simulink model "parallel_8_prediction"  (R2022a)
settings: Solver=FixedStepDiscrete  StartTime=0.0  StopTime=10.0  RelTol=1e-3
undefined symbols (not defined in the file or in its folder): f_c, L_d, L_q, L_x, L_y, p, psi_pm, R_ph
libraries: hdlsllib x5
(part 1 of 2)
settings Model: DataTypeOverride=Off  Creator=Andre Merx  LastModifiedBy=Andre Merx
settings SolverCC: AlgebraicLoopSolver=TrustRegion
settings DataIOCC: LimitDataPoints=on  SaveOutput=off  SaveTime=off
settings OptimizationCC: BlockReduction=off  ConditionallyExecuteInputs=off  DefaultParameterBehavior=Inlined  LifeSpan=inf
settings DebuggingCC: AlgebraicLoopMsg=error  SingleTaskRateTransMsg=error  UnconnectedInputMsg=warning  UnconnectedOutputMsg=warning  UnconnectedLineMsg=warning  AllowSymbolicDim=off  StrictBusMsg=ErrorOnBusTreatedAsVector  SFUnexpectedBacktrackingDiag=warning  SFNoUnconditionalDefaultTransitionDiag=warning  SFExecutionAtInitializationDiag=none  SFMachineParentedDataDiag=warning  ArithmeticOperatorsInVariantConditions=warning
settings HardwareCC: ProdBitPerPointer=32  ProdBitPerSizeT=32  ProdBitPerPtrDiffT=32  ProdLargestAtomicFloat=None  ProdIntDivRoundTo=Undefined  ProdEndianess=Unspecified  ProdWordSize=32  ProdHWDeviceType=ASIC/FPGA->ASIC/FPGA  ProdEqTarget=off
settings SFSimCC: SimUseLocalCustomCode=off  CustomCodeUndefinedFunction=UseInterfaceOnly
settings RTWCC: RTWUseLocalCustomCode=off
settings CodeAppCC: StateflowObjectComments=on
settings GRTTargetCC: TargetLangStandard=C89/C90 (ANSI)
settings ConfigComp: CovScope=ReferencedModels  CovMetricSettings=dw  CovSaveCumulativeToWorkspaceVar=on  CovSaveSingleToWorkspaceVar=on  CovExternalEMLEnable=off  CovSFcnEnable=off

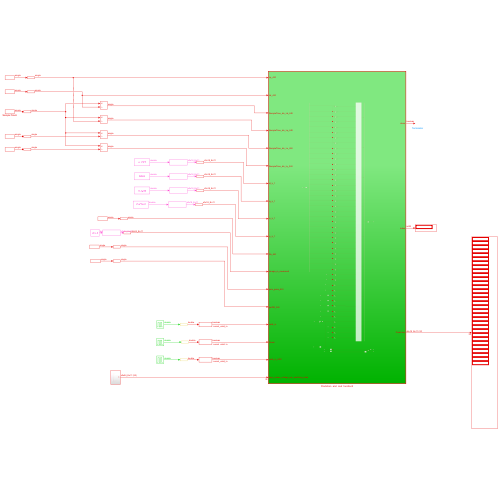
[thumbnail: Simulink's stored preview of the top-level diagram]
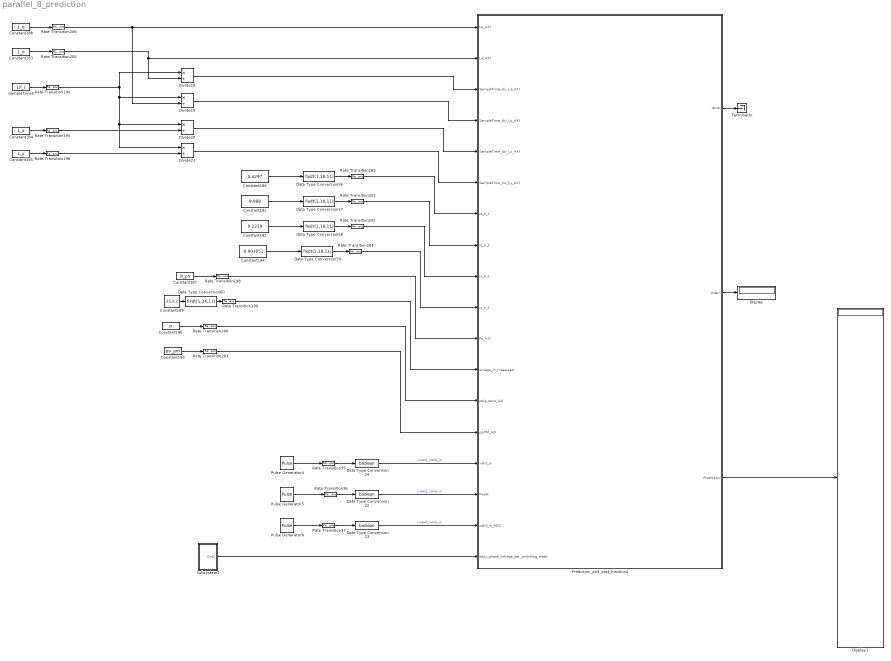
== system parallel_8_prediction ==
  Constant183 : Constant  Value=L_d  OutDataTypeStr=single  SampleTime=-1
  Constant184 : Constant  Value=L_x  OutDataTypeStr=single  SampleTime=-1
  Constant185 : Constant  Value=L_y  OutDataTypeStr=single  SampleTime=-1
  Constant186 : Constant  Value=0.4297
  Constant187 : Constant  Value=R_ph  OutDataTypeStr=single  SampleTime=-1
  Constant188 : Constant  Value=L_q  OutDataTypeStr=single  SampleTime=-1
  Constant189 : Constant  Value=313.3
  Constant190 : Constant  Value=p  OutDataTypeStr=single  SampleTime=-1
  Constant191 : Constant  Value=9.988
  Constant192 : Constant  Value=0.2219
  Constant193 : Constant  Value=psi_pm  OutDataTypeStr=single  SampleTime=-1
  Constant194 : Constant  Value=-0.003051
  Data Type Conversion22 : DataTypeConversion  OutDataTypeStr=boolean  SaturateOnIntegerOverflow=off  RndMeth=Floor
  Data Type Conversion23 : DataTypeConversion  OutDataTypeStr=boolean  SaturateOnIntegerOverflow=off  RndMeth=Floor
  Data Type Conversion24 : DataTypeConversion  OutDataTypeStr=boolean  SaturateOnIntegerOverflow=off  RndMeth=Floor
  Data Type Conversion{56..59} (4 alike) : DataTypeConversion  OutDataTypeStr=fixdt(1,18,11)  SaturateOnIntegerOverflow=off  RndMeth=Floor
  Data Type Conversion60 : DataTypeConversion  OutDataTypeStr=fixdt(1,24,11)  SaturateOnIntegerOverflow=off  RndMeth=Floor
  Display : Display
  Display1 : Display
  Divide{18..21} (4 alike) : Product  Inputs=*/  RndMeth=Zero  SaturateOnIntegerOverflow=on
  Prediction_and_cost_function2 : Subsystem  TreatAsAtomicUnit=on
  Pulse Generator4 : DiscretePulseGenerator  PulseType=Time based  Period=1/f_c
  Pulse Generator5 : DiscretePulseGenerator  PulseType=Time based  Period=1/f_c
  Pulse Generator6 : DiscretePulseGenerator  PulseType=Time based  Period=1/f_c
  Rate Transition{35..37,193..196,198..206} (16 alike) : RateTransition  OutPortSampleTime=Rt
  SampleTime5 : Constant  Value=1/f_c  OutDataTypeStr=single  SampleTime=-1
  Subsystem2 : Subsystem
  Terminator : Terminator
  wires:
  Data Type Conversion60/1 -> Rate Transition199/1
  Rate Transition199/1 -> Prediction_and_cost_function2/12(omega_m_measured)
  Constant194/1 -> Data Type Conversion59/1
  Constant188/1 -> Rate Transition206/1
  Rate Transition201/1 -> Prediction_and_cost_function2/8(iq_k_1)
  Data Type Conversion59/1 -> Rate Transition204/1
  Constant190/1 -> Rate Transition200/1
  Subsystem2/1(Out1) -> Prediction_and_cost_function2/18(dqxy_phase_voltage_per_switching_state)
  Rate Transition205/1 -> Divide18/2, Prediction_and_cost_function2/2(Ld_AXI)
  Data Type Conversion58/1 -> Rate Transition202/1
  Rate Transition195/1 -> Divide20/2
  SampleTime5/1 -> Rate Transition194/1
  Constant186/1 -> Data Type Conversion56/1
  Data Type Conversion57/1 -> Rate Transition201/1
  Divide20/1 -> Prediction_and_cost_function2/5(SampleTime_div_Lx_AXI)
  Constant187/1 -> Rate Transition198/1
  Rate Transition203/1 -> Prediction_and_cost_function2/14(psiPM_AXI)
  Data Type Conversion56/1 -> Rate Transition193/1
  Constant192/1 -> Data Type Conversion58/1
  Rate Transition196/1 -> Divide21/2
  Divide19/1 -> Prediction_and_cost_function2/4(SampleTime_div_Lq_AXI)
  Rate Transition206/1 -> Divide19/2, Prediction_and_cost_function2/1(Lq_AXI)
  Rate Transition200/1 -> Prediction_and_cost_function2/13(pole_pairs_AXI)
  Constant193/1 -> Rate Transition203/1
  Constant184/1 -> Rate Transition195/1
  Constant183/1 -> Rate Transition205/1
  Constant189/1 -> Data Type Conversion60/1
  Divide21/1 -> Prediction_and_cost_function2/6(SampleTime_div_Ly_AXI)
  Rate Transition202/1 -> Prediction_and_cost_function2/9(ix_k_1)
  Constant185/1 -> Rate Transition196/1
  Constant191/1 -> Data Type Conversion57/1
  Divide18/1 -> Prediction_and_cost_function2/3(SampleTime_div_Ld_AXI)
  Rate Transition198/1 -> Prediction_and_cost_function2/11(Rs_AXI)
  Rate Transition194/1 -> Divide19/1, Divide21/1, Divide20/1, Divide18/1
  Rate Transition193/1 -> Prediction_and_cost_function2/7(id_k_1)
  Rate Transition204/1 -> Prediction_and_cost_function2/10(iy_k_1)
  Pulse Generator4/1 -> Rate Transition35/1
  Rate Transition36/1 -> Data Type Conversion22/1
  Data Type Conversion23/1 -> Prediction_and_cost_function2/17(valid_in_ADC)  "curent_valid_in"
  Rate Transition35/1 -> Data Type Conversion24/1
  Rate Transition37/1 -> Data Type Conversion23/1
  Data Type Conversion24/1 -> Prediction_and_cost_function2/15(valid_in)  "curent_valid_in"
  Data Type Conversion22/1 -> Prediction_and_cost_function2/16(Reset)  "curent_valid_in"
  Pulse Generator6/1 -> Rate Transition37/1
  Pulse Generator5/1 -> Rate Transition36/1
  Prediction_and_cost_function2/1(done) -> Terminator/1
  Prediction_and_cost_function2/2(Index) -> Display/1
  Prediction_and_cost_function2/3(Prediction) -> Display1/1

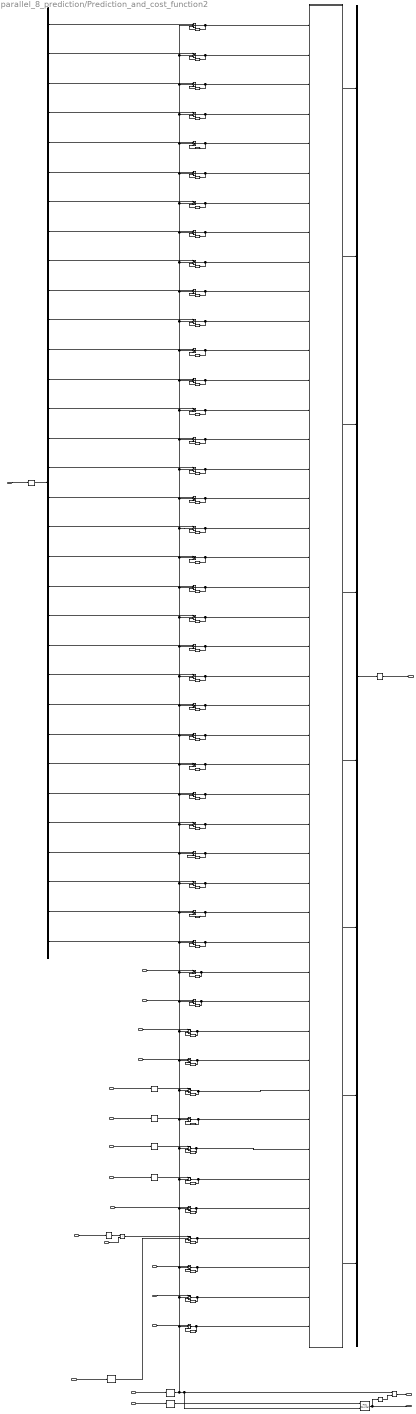
== system parallel_8_prediction/Prediction_and_cost_function2 ==
  Lq_AXI : Inport
  Ld_AXI : Inport  Port=2
  SampleTime_div_Ld_AXI : Inport  Port=3
  SampleTime_div_Lq_AXI : Inport  Port=4
  SampleTime_div_Lx_AXI : Inport  Port=5
  SampleTime_div_Ly_AXI : Inport  Port=6
  id_k_1 : Inport  Port=7
  iq_k_1 : Inport  Port=8
  ix_k_1 : Inport  Port=9
  iy_k_1 : Inport  Port=10
  Rs_AXI : Inport  Port=11
  omega_m_measured : Inport  Port=12
  pole_pairs_AXI : Inport  Port=13
  psiPM_AXI : Inport  Port=14
  valid_in : Inport  Port=15
  Reset : Inport  Port=16
  valid_in_ADC : Inport  Port=17
  dqxy_phase_voltage_per_switching_state : Inport  Port=18
  Compare To Constant : hdlsllib/Logic and Bit Operations/Compare To Constant  relop=<=  const=8  OutDataTypeStr=boolean
      settings: SourceProductBaseCode=SL
  Data Type Conversion{1,4,7..10} (6 alike) : DataTypeConversion  OutDataTypeStr=single  RndMeth=Nearest  SaturateOnIntegerOverflow=off
  Data Type Conversion18 : DataTypeConversion  OutDataTypeStr=fixdt(1,18,11)  RndMeth=Nearest  SaturateOnIntegerOverflow=off
  Delay{8..20,104..135} (45 alike) : Delay  DelayLength=1
  Demux : Demux  Outputs=32
  Detect Rise Positive : hdlsllib/Logic and Bit Operations/Detect Rise Positive  vinit=0  OutDataTypeStr=boolean
      settings: SourceProductBaseCode=SL
  Detect Rise Positive1 : hdlsllib/Logic and Bit Operations/Detect Rise Positive  vinit=0  OutDataTypeStr=boolean
      settings: SourceProductBaseCode=SL
  Detect Rise Positive2 : hdlsllib/Logic and Bit Operations/Detect Rise Positive  vinit=0  OutDataTypeStr=boolean
      settings: SourceProductBaseCode=SL
  HDL Counter : hdlsllib/Sources/HDL Counter  CountType=Free running  CountInit=0  CountStep=1  CountMax=25  CountFromType=Initial value  CountFrom=0  CountResetPort=on  CountLoadPort=off  CountEnbPort=on  CountDirPort=off  CountHitOutputPort=off  CountDataType=Signed  CountWordLen=32  CountFracLen=0  CountSampTime=1
  Logical Operator : Logic  AllPortsSameDT=off  OutDataTypeStr=boolean
  Mux : Mux  Inputs=8
  Product : Product  Inputs=**
  Subsystem : Subsystem
  Switch_on{8..13,15..21,59..90} (45 alike) : Switch  Threshold=1  OutDataTypeStr=single  RndMeth=Simplest  SaturateOnIntegerOverflow=off  InputSameDT=off
  done : Outport
  Index : Outport  Port=2
  Prediction : Outport  Port=3
  wires:
  Switch_on12/1 -> Subsystem/41(Rs15), Delay12/1
  Rs_AXI/1 -> Switch_on12/1
  SampleTime_div_Ld_AXI/1 -> Switch_on21/1
  Delay10/1 -> Switch_on10/3
  Delay17/1 -> Switch_on18/3
  Switch_on10/1 -> Delay10/1, Subsystem/43(Lq15)
  Delay11/1 -> Switch_on11/3
  SampleTime_div_Lq_AXI/1 -> Switch_on20/1
  Ld_AXI/1 -> Switch_on9/1
  psiPM_AXI/1 -> Switch_on8/1
  Product/1 -> Switch_on11/1  "omega_el"
  Delay9/1 -> Switch_on9/3
  Data Type Conversion4/1 -> Product/1
  Delay20/1 -> Switch_on21/3
  pole_pairs_AXI/1 -> Product/2
  Switch_on18/1 -> Delay17/1, Subsystem/36(SampleTime_div_Ly15)
  Delay19/1 -> Switch_on20/3
  Delay13/1 -> Switch_on13/3
  Switch_on15/1 -> Delay14/1, Subsystem/39(ix_k_16)
  Delay18/1 -> Switch_on19/3
  Switch_on19/1 -> Delay18/1, Subsystem/35(SampleTime_div_Lx15)
  Switch_on20/1 -> Delay19/1, Subsystem/34(SampleTime_div_Lq15)
  Switch_on13/1 -> Delay13/1, Subsystem/40(iy_k_16)
  Delay16/1 -> Switch_on17/3
  Switch_on17/1 -> Delay16/1, Subsystem/37(id_k_16)
  Delay15/1 -> Switch_on16/3
  Switch_on16/1 -> Delay15/1, Subsystem/38(iq_k_16)
  Switch_on11/1 -> Delay11/1, Subsystem/42(omega_el15)
  SampleTime_div_Lx_AXI/1 -> Switch_on19/1
  Delay12/1 -> Switch_on12/3
  Switch_on21/1 -> Delay20/1, Subsystem/33(SampleTime_div_Ld15)
  Lq_AXI/1 -> Switch_on10/1
  Switch_on9/1 -> Delay9/1, Subsystem/44(Ld15)
  SampleTime_div_Ly_AXI/1 -> Switch_on18/1
  Delay14/1 -> Switch_on15/3
  Switch_on8/1 -> Delay8/1, Subsystem/45(psiPM15)
  Delay8/1 -> Switch_on8/3
  id_k_1/1 -> Data Type Conversion7/1
  iq_k_1/1 -> Data Type Conversion8/1
  ix_k_1/1 -> Data Type Conversion9/1
  iy_k_1/1 -> Data Type Conversion10/1
  omega_m_measured/1 -> Data Type Conversion4/1
  Data Type Conversion7/1 -> Switch_on17/1
  Data Type Conversion8/1 -> Switch_on16/1
  Data Type Conversion9/1 -> Switch_on15/1
  Data Type Conversion10/1 -> Switch_on13/1
  Detect Rise Positive1/1 -> HDL Counter/1  "reset"
  Compare To Constant/1 -> Logical Operator/2
  Detect Rise Positive2/1 -> Switch_on11/2  "End_Cycle"
  Data Type Conversion18/1 -> Prediction/1
  Switch_on61/1 -> Subsystem/30(q_phase_voltage_per_switching_state7), Delay106/1
  Delay106/1 -> Switch_on61/3
  Delay107/1 -> Switch_on62/3
  Switch_on62/1 -> Delay107/1, Subsystem/29(d_phase_voltage_per_switching_state7)
  Delay104/1 -> Switch_on59/3
  Switch_on59/1 -> Delay104/1, Subsystem/32(y_phase_voltage_per_switching_state7)
  Delay105/1 -> Switch_on60/3
  Switch_on60/1 -> Subsystem/31(x_phase_voltage_per_switching_state7), Delay105/1
  Switch_on65/1 -> Subsystem/26(q_phase_voltage_per_switching_state6), Delay110/1
  Delay110/1 -> Switch_on65/3
  Delay111/1 -> Switch_on66/3
  Switch_on66/1 -> Subsystem/25(d_phase_voltage_per_switching_state6), Delay111/1
  Delay108/1 -> Switch_on63/3
  Switch_on63/1 -> Subsystem/28(y_phase_voltage_per_switching_state6), Delay108/1
  Delay109/1 -> Switch_on64/3
  Switch_on64/1 -> Subsystem/27(x_phase_voltage_per_switching_state6), Delay109/1
  Switch_on69/1 -> Subsystem/22(q_phase_voltage_per_switching_state5), Delay114/1
  Delay114/1 -> Switch_on69/3
  Delay115/1 -> Switch_on70/3
  Switch_on70/1 -> Subsystem/21(d_phase_voltage_per_switching_state5), Delay115/1
  Delay112/1 -> Switch_on67/3
  Switch_on67/1 -> Subsystem/24(y_phase_voltage_per_switching_state5), Delay112/1
  Delay113/1 -> Switch_on68/3
  Switch_on68/1 -> Subsystem/23(x_phase_voltage_per_switching_state5), Delay113/1
  Switch_on73/1 -> Subsystem/18(q_phase_voltage_per_switching_state4), Delay118/1
  Delay118/1 -> Switch_on73/3
  Delay119/1 -> Switch_on74/3
  Switch_on74/1 -> Subsystem/17(d_phase_voltage_per_switching_state4), Delay119/1
  Delay116/1 -> Switch_on71/3
  Switch_on71/1 -> Subsystem/20(y_phase_voltage_per_switching_state4), Delay116/1
  Delay117/1 -> Switch_on72/3
  Switch_on72/1 -> Subsystem/19(x_phase_voltage_per_switching_state4), Delay117/1
  Switch_on77/1 -> Subsystem/14(q_phase_voltage_per_switching_state3), Delay122/1
  Delay122/1 -> Switch_on77/3
  Delay123/1 -> Switch_on78/3
  Switch_on78/1 -> Subsystem/13(d_phase_voltage_per_switching_state3), Delay123/1
  Delay120/1 -> Switch_on75/3
  Switch_on75/1 -> Subsystem/16(y_phase_voltage_per_switching_state3), Delay120/1
  Delay121/1 -> Switch_on76/3
  Switch_on76/1 -> Subsystem/15(x_phase_voltage_per_switching_state3), Delay121/1
  Switch_on81/1 -> Subsystem/10(q_phase_voltage_per_switching_state2), Delay126/1
  Delay126/1 -> Switch_on81/3
  Delay127/1 -> Switch_on82/3
  Switch_on82/1 -> Subsystem/9(d_phase_voltage_per_switching_state2), Delay127/1
  Delay124/1 -> Switch_on79/3
  Switch_on79/1 -> Subsystem/12(y_phase_voltage_per_switching_state2), Delay124/1
  Delay125/1 -> Switch_on80/3
  Switch_on80/1 -> Subsystem/11(x_phase_voltage_per_switching_state2), Delay125/1
  Switch_on85/1 -> Subsystem/6(q_phase_voltage_per_switching_state1), Delay130/1
  Delay130/1 -> Switch_on85/3
  Delay131/1 -> Switch_on86/3
  Switch_on86/1 -> Subsystem/5(d_phase_voltage_per_switching_state1), Delay131/1
  Delay128/1 -> Switch_on83/3
  Switch_on83/1 -> Subsystem/8(y_phase_voltage_per_switching_state1), Delay128/1
  Delay129/1 -> Switch_on84/3
  Switch_on84/1 -> Subsystem/7(x_phase_voltage_per_switching_state1), Delay129/1
  Switch_on89/1 -> Subsystem/2(q_phase_voltage_per_switching_state), Delay134/1
  Delay134/1 -> Switch_on89/3
  Delay135/1 -> Switch_on90/3
  Switch_on90/1 -> Subsystem/1(d_phase_voltage_per_switching_state), Delay135/1
  Delay132/1 -> Switch_on87/3
  Switch_on87/1 -> Subsystem/4(y_phase_voltage_per_switching_state), Delay132/1
  Delay133/1 -> Switch_on88/3
  Switch_on88/1 -> Subsystem/3(x_phase_voltage_per_switching_state), Delay133/1
  Detect Rise Positive/1 -> HDL Counter/2, Logical Operator/1, Switch_on8/2, Switch_on9/2, Switch_on10/2, Switch_on16/2, Switch_on18/2, Switch_on19/2, Switch_on20/2, Switch_on21/2, Switch_on59/2, Switch_on60/2, Switch_on61/2, Switch_on62/2, Switch_on63/2, Switch_on64/2, Switch_on65/2, Switch_on66/2, Switch_on67/2, Switch_on68/2, Switch_on69/2, Switch_on70/2, Switch_on71/2, Switch_on72/2, Switch_on73/2, Switch_on74/2, Switch_on75/2, Switch_on76/2, Switch_on77/2, Switch_on78/2, Switch_on79/2, Switch_on80/2, Switch_on81/2, Switch_on82/2, Switch_on83/2, Switch_on84/2, Switch_on85/2, Switch_on86/2, Switch_on87/2, Switch_on88/2, Switch_on89/2, Switch_on90/2, Switch_on17/2, Switch_on15/2, Switch_on13/2, Switch_on12/2  "enable"
  Demux/32 -> Switch_on59/1
  Demux/31 -> Switch_on60/1
  Demux/30 -> Switch_on61/1
  Demux/29 -> Switch_on62/1
  Demux/28 -> Switch_on63/1
  Demux/27 -> Switch_on64/1
  Demux/26 -> Switch_on65/1
  Demux/25 -> Switch_on66/1
  Demux/24 -> Switch_on67/1
  Demux/23 -> Switch_on68/1
  Demux/22 -> Switch_on69/1
  Demux/21 -> Switch_on70/1
  Demux/20 -> Switch_on71/1
  Demux/19 -> Switch_on72/1
  Demux/18 -> Switch_on73/1
  Demux/17 -> Switch_on74/1
  Demux/16 -> Switch_on75/1
  Demux/15 -> Switch_on76/1
  Demux/14 -> Switch_on77/1
  Demux/13 -> Switch_on78/1
  Demux/12 -> Switch_on79/1
  Demux/11 -> Switch_on80/1
  Demux/10 -> Switch_on81/1
  Demux/9 -> Switch_on82/1
  Demux/8 -> Switch_on83/1
  Demux/7 -> Switch_on84/1
  Demux/6 -> Switch_on85/1
  Demux/5 -> Switch_on86/1
  Demux/4 -> Switch_on87/1
  Demux/3 -> Switch_on88/1
  Demux/2 -> Switch_on89/1
  Demux/1 -> Switch_on90/1
  Subsystem/8(Prediction_8) -> Mux/8
  Subsystem/7(Prediction_7) -> Mux/7
  Subsystem/6(Prediction_6) -> Mux/6
  Subsystem/5(Prediction_5) -> Mux/5
  Subsystem/4(Prediction_4) -> Mux/4
  Subsystem/3(Prediction_3) -> Mux/3
  Subsystem/2(Prediction_2) -> Mux/2
  Subsystem/1(Prediction_1) -> Mux/1
  Mux/1 -> Data Type Conversion18/1
  dqxy_phase_voltage_per_switching_state/1 -> Data Type Conversion1/1
  Data Type Conversion1/1 -> Demux/1
  HDL Counter/1 -> Index/1, Compare To Constant/1  "Index"
  valid_in_ADC/1 -> Detect Rise Positive2/1
  valid_in/1 -> Detect Rise Positive/1
  Reset/1 -> Detect Rise Positive1/1
  Logical Operator/1 -> done/1

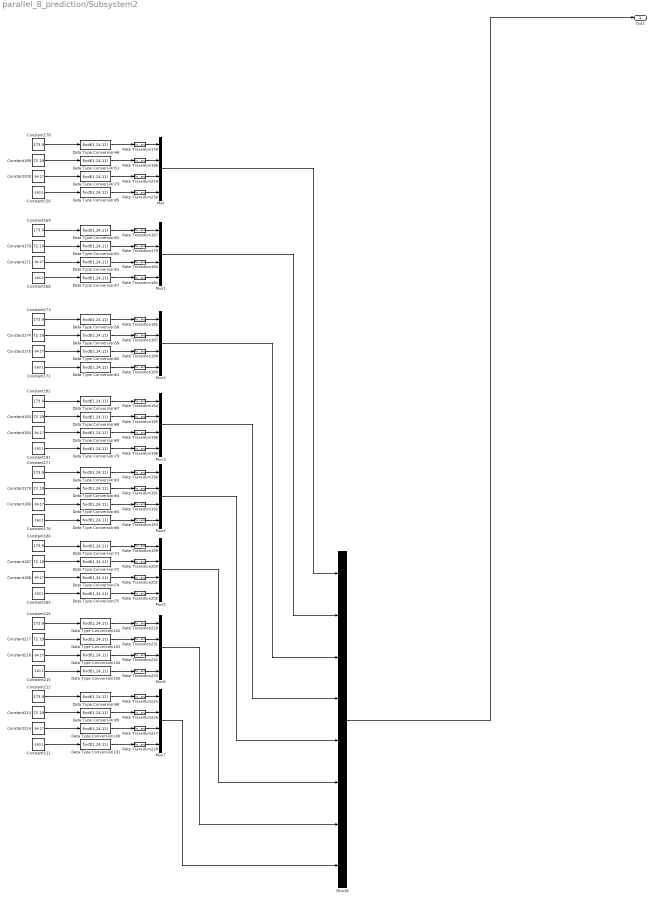
== system parallel_8_prediction/Subsystem2 ==
  Constant{156,168,172,176,181,185,211,215} (8 alike) : Constant  Value=-163.1
  Constant{169,173,177..178,182,186,212,216} (8 alike) : Constant  Value=173.9
  Constant{170,174,179,183,187,189,213,217} (8 alike) : Constant  Value=72.19
  Constant{171,175,180,184,188,200,214,218} (8 alike) : Constant  Value=-94.17
  Data Type Conversion{46,51..53,57..75,95,98..105} (32 alike) : DataTypeConversion  OutDataTypeStr=fixdt(1,24,11)  SaturateOnIntegerOverflow=off  RndMeth=Floor
  Mux{,1..7} (8 alike) : Mux
  Mux16 : Mux  Inputs=8
  Rate Transition{167,178..180,184..196,198..202,219,225..233} (32 alike) : RateTransition  OutPortSampleTime=Rt
  Out1 : Outport
  wires:
  Constant169/1 -> Data Type Conversion62/1
  Data Type Conversion95/1 -> Rate Transition230/1
  Rate Transition201/1 -> Mux5/3
  Data Type Conversion103/1 -> Rate Transition231/1
  Data Type Conversion60/1 -> Rate Transition188/1
  Rate Transition187/1 -> Mux2/2
  Data Type Conversion58/1 -> Rate Transition185/1
  Data Type Conversion64/1 -> Rate Transition191/1
  Rate Transition180/1 -> Mux1/3
  Mux3/1 -> Mux16/4
  Rate Transition199/1 -> Mux5/1
  Data Type Conversion71/1 -> Rate Transition199/1
  Data Type Conversion51/1 -> Rate Transition186/1
  Constant187/1 -> Data Type Conversion72/1
  Data Type Conversion99/1 -> Rate Transition226/1
  Rate Transition191/1 -> Mux4/2
  Mux2/1 -> Mux16/3
  Constant179/1 -> Data Type Conversion64/1
  Constant200/1 -> Data Type Conversion73/1
  Constant188/1 -> Data Type Conversion74/1
  Rate Transition229/1 -> Mux6/1
  Rate Transition194/1 -> Mux3/1
  Mux5/1 -> Mux16/6
  Constant180/1 -> Data Type Conversion65/1
  Rate Transition188/1 -> Mux2/3
  Rate Transition233/1 -> Mux6/4
  Rate Transition202/1 -> Mux5/4
  Constant181/1 -> Data Type Conversion70/1
  Constant212/1 -> Data Type Conversion98/1
  Rate Transition193/1 -> Mux4/4
  Rate Transition186/1 -> Mux/2
  Rate Transition232/1 -> Mux6/3
  Data Type Conversion53/1 -> Rate Transition180/1
  Mux6/1 -> Mux16/7
  Constant178/1 -> Data Type Conversion46/1
  Data Type Conversion68/1 -> Rate Transition195/1
  Mux/1 -> Mux16/1
  Constant215/1 -> Data Type Conversion105/1
  Mux1/1 -> Mux16/2
  Rate Transition227/1 -> Mux7/3
  Constant171/1 -> Data Type Conversion53/1
  Data Type Conversion69/1 -> Rate Transition196/1
  Rate Transition228/1 -> Mux7/4
  Constant214/1 -> Data Type Conversion100/1
  Constant216/1 -> Data Type Conversion102/1
  Constant185/1 -> Data Type Conversion75/1
  Data Type Conversion52/1 -> Rate Transition179/1
  Mux4/1 -> Mux16/5
  Rate Transition178/1 -> Mux/1
  Data Type Conversion98/1 -> Rate Transition225/1
  Constant186/1 -> Data Type Conversion71/1
  Data Type Conversion66/1 -> Rate Transition193/1
  Mux7/1 -> Mux16/8
  Rate Transition225/1 -> Mux7/1
  Constant175/1 -> Data Type Conversion60/1
  Data Type Conversion62/1 -> Rate Transition167/1
  Rate Transition179/1 -> Mux1/2
  Data Type Conversion101/1 -> Rate Transition228/1
  Constant168/1 -> Data Type Conversion57/1
  Data Type Conversion63/1 -> Rate Transition190/1
  Data Type Conversion46/1 -> Rate Transition178/1
  Constant213/1 -> Data Type Conversion99/1
  Constant211/1 -> Data Type Conversion101/1
  Rate Transition226/1 -> Mux7/2
  Rate Transition189/1 -> Mux2/4
  Constant173/1 -> Data Type Conversion58/1
  Rate Transition231/1 -> Mux6/2
  Data Type Conversion61/1 -> Rate Transition189/1
  Data Type Conversion57/1 -> Rate Transition184/1
  Constant172/1 -> Data Type Conversion61/1
  Data Type Conversion59/1 -> Rate Transition187/1
  Constant189/1 -> Data Type Conversion51/1
  Data Type Conversion75/1 -> Rate Transition202/1
  Constant182/1 -> Data Type Conversion67/1
  Data Type Conversion70/1 -> Rate Transition198/1
  Rate Transition184/1 -> Mux1/4
  Constant184/1 -> Data Type Conversion69/1
  Data Type Conversion73/1 -> Rate Transition219/1
  Data Type Conversion67/1 -> Rate Transition194/1
  Rate Transition195/1 -> Mux3/2
  Constant170/1 -> Data Type Conversion52/1
  Rate Transition190/1 -> Mux4/1
  Rate Transition192/1 -> Mux4/3
  Rate Transition200/1 -> Mux5/2
  Rate Transition198/1 -> Mux3/4
  Constant156/1 -> Data Type Conversion95/1
  Data Type Conversion102/1 -> Rate Transition229/1
  Rate Transition219/1 -> Mux/3
  Rate Transition167/1 -> Mux1/1
  Rate Transition230/1 -> Mux/4
  Rate Transition196/1 -> Mux3/3
  Rate Transition185/1 -> Mux2/1
  Constant174/1 -> Data Type Conversion59/1
  Data Type Conversion72/1 -> Rate Transition200/1
  Constant217/1 -> Data Type Conversion103/1
  Data Type Conversion104/1 -> Rate Transition232/1
  Data Type Conversion105/1 -> Rate Transition233/1
  Data Type Conversion74/1 -> Rate Transition201/1
  Constant176/1 -> Data Type Conversion66/1
  Constant183/1 -> Data Type Conversion68/1
  Constant177/1 -> Data Type Conversion63/1
  Constant218/1 -> Data Type Conversion104/1
  Data Type Conversion100/1 -> Rate Transition227/1
  Data Type Conversion65/1 -> Rate Transition192/1
  Mux16/1 -> Out1/1

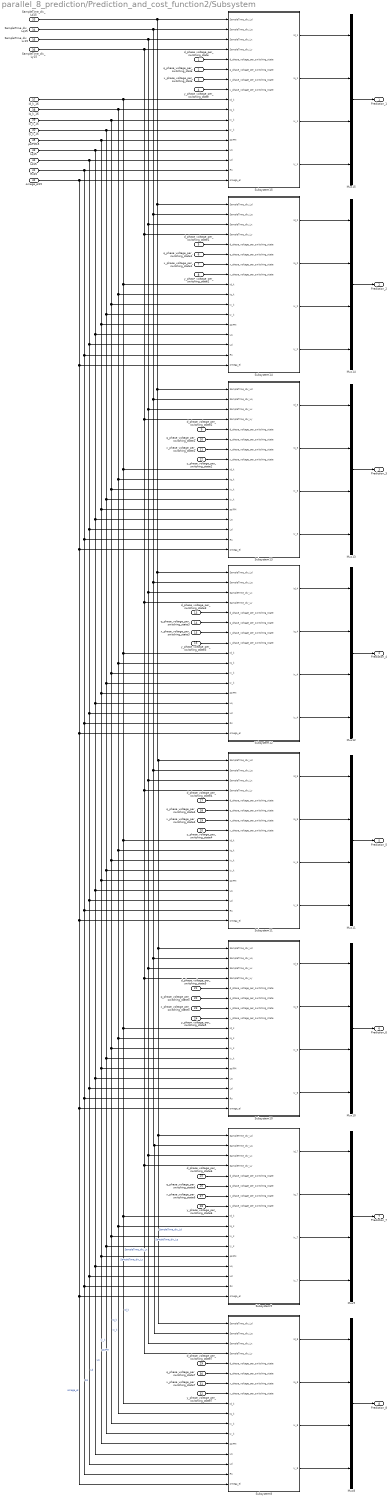
== system parallel_8_prediction/Prediction_and_cost_function2/Subsystem ==
  d_phase_voltage_per_switching_state : Inport
  q_phase_voltage_per_switching_state : Inport  Port=2
  x_phase_voltage_per_switching_state : Inport  Port=3
  y_phase_voltage_per_switching_state : Inport  Port=4
  d_phase_voltage_per_switching_state1 : Inport  Port=5
  q_phase_voltage_per_switching_state1 : Inport  Port=6
  x_phase_voltage_per_switching_state1 : Inport  Port=7
  y_phase_voltage_per_switching_state1 : Inport  Port=8
  d_phase_voltage_per_switching_state2 : Inport  Port=9
  q_phase_voltage_per_switching_state2 : Inport  Port=10
  x_phase_voltage_per_switching_state2 : Inport  Port=11
  y_phase_voltage_per_switching_state2 : Inport  Port=12
  d_phase_voltage_per_switching_state3 : Inport  Port=13
  q_phase_voltage_per_switching_state3 : Inport  Port=14
  x_phase_voltage_per_switching_state3 : Inport  Port=15
  y_phase_voltage_per_switching_state3 : Inport  Port=16
  d_phase_voltage_per_switching_state4 : Inport  Port=17
  q_phase_voltage_per_switching_state4 : Inport  Port=18
  x_phase_voltage_per_switching_state4 : Inport  Port=19
  y_phase_voltage_per_switching_state4 : Inport  Port=20
  d_phase_voltage_per_switching_state5 : Inport  Port=21
  q_phase_voltage_per_switching_state5 : Inport  Port=22
  x_phase_voltage_per_switching_state5 : Inport  Port=23
  y_phase_voltage_per_switching_state5 : Inport  Port=24
  d_phase_voltage_per_switching_state6 : Inport  Port=25
  q_phase_voltage_per_switching_state6 : Inport  Port=26
  x_phase_voltage_per_switching_state6 : Inport  Port=27
  y_phase_voltage_per_switching_state6 : Inport  Port=28
  d_phase_voltage_per_switching_state7 : Inport  Port=29
  q_phase_voltage_per_switching_state7 : Inport  Port=30
  x_phase_voltage_per_switching_state7 : Inport  Port=31
  y_phase_voltage_per_switching_state7 : Inport  Port=32
  SampleTime_div_Ld15 : Inport  Port=33
  SampleTime_div_Lq15 : Inport  Port=34
  SampleTime_div_Lx15 : Inport  Port=35
  SampleTime_div_Ly15 : Inport  Port=36
  id_k_16 : Inport  Port=37
  iq_k_16 : Inport  Port=38
  ix_k_16 : Inport  Port=39
  iy_k_16 : Inport  Port=40
  Rs15 : Inport  Port=41
  omega_el15 : Inport  Port=42
  Lq15 : Inport  Port=43
  Ld15 : Inport  Port=44
  psiPM15 : Inport  Port=45
  Mux{8..15} (8 alike) : Mux
  Subsystem10 : Subsystem
  Subsystem11 : Subsystem
  Subsystem12 : Subsystem
  Subsystem13 : Subsystem
  Subsystem14 : Subsystem
  Subsystem15 : Subsystem
  Subsystem8 : Subsystem
  Subsystem9 : Subsystem
  Prediction_1 : Outport
  Prediction_2 : Outport  Port=2
  Prediction_3 : Outport  Port=3
  Prediction_4 : Outport  Port=4
  Prediction_5 : Outport  Port=5
  Prediction_6 : Outport  Port=6
  Prediction_7 : Outport  Port=7
  Prediction_8 : Outport  Port=8
  wires:
  q_phase_voltage_per_switching_state1/1 -> Subsystem14/6(q_phase_voltage_per_switching_state)
  y_phase_voltage_per_switching_state/1 -> Subsystem15/8(y_phase_voltage_per_switching_state)
  y_phase_voltage_per_switching_state2/1 -> Subsystem13/8(y_phase_voltage_per_switching_state)
  d_phase_voltage_per_switching_state1/1 -> Subsystem14/5(d_phase_voltage_per_switching_state)
  x_phase_voltage_per_switching_state1/1 -> Subsystem14/7(x_phase_voltage_per_switching_state)
  y_phase_voltage_per_switching_state7/1 -> Subsystem8/8(y_phase_voltage_per_switching_state)
  d_phase_voltage_per_switching_state3/1 -> Subsystem12/5(d_phase_voltage_per_switching_state)
  d_phase_voltage_per_switching_state6/1 -> Subsystem9/5(d_phase_voltage_per_switching_state)
  d_phase_voltage_per_switching_state/1 -> Subsystem15/5(d_phase_voltage_per_switching_state)
  x_phase_voltage_per_switching_state3/1 -> Subsystem12/7(x_phase_voltage_per_switching_state)
  d_phase_voltage_per_switching_state2/1 -> Subsystem13/5(d_phase_voltage_per_switching_state)
  x_phase_voltage_per_switching_state4/1 -> Subsystem11/7(x_phase_voltage_per_switching_state)
  y_phase_voltage_per_switching_state1/1 -> Subsystem14/8(y_phase_voltage_per_switching_state)
  q_phase_voltage_per_switching_state2/1 -> Subsystem13/6(q_phase_voltage_per_switching_state)
  x_phase_voltage_per_switching_state2/1 -> Subsystem13/7(x_phase_voltage_per_switching_state)
  y_phase_voltage_per_switching_state4/1 -> Subsystem11/8(y_phase_voltage_per_switching_state)
  x_phase_voltage_per_switching_state/1 -> Subsystem15/7(x_phase_voltage_per_switching_state)
  q_phase_voltage_per_switching_state5/1 -> Subsystem10/6(q_phase_voltage_per_switching_state)
  d_phase_voltage_per_switching_state7/1 -> Subsystem8/5(d_phase_voltage_per_switching_state)
  d_phase_voltage_per_switching_state4/1 -> Subsystem11/5(d_phase_voltage_per_switching_state)
  q_phase_voltage_per_switching_state4/1 -> Subsystem11/6(q_phase_voltage_per_switching_state)
  x_phase_voltage_per_switching_state5/1 -> Subsystem10/7(x_phase_voltage_per_switching_state)
  x_phase_voltage_per_switching_state7/1 -> Subsystem8/7(x_phase_voltage_per_switching_state)
  q_phase_voltage_per_switching_state/1 -> Subsystem15/6(q_phase_voltage_per_switching_state)
  d_phase_voltage_per_switching_state5/1 -> Subsystem10/5(d_phase_voltage_per_switching_state)
  y_phase_voltage_per_switching_state5/1 -> Subsystem10/8(y_phase_voltage_per_switching_state)
  q_phase_voltage_per_switching_state6/1 -> Subsystem9/6(q_phase_voltage_per_switching_state)
  y_phase_voltage_per_switching_state6/1 -> Subsystem9/8(y_phase_voltage_per_switching_state)
  x_phase_voltage_per_switching_state6/1 -> Subsystem9/7(x_phase_voltage_per_switching_state)
  q_phase_voltage_per_switching_state7/1 -> Subsystem8/6(q_phase_voltage_per_switching_state)
  y_phase_voltage_per_switching_state3/1 -> Subsystem12/8(y_phase_voltage_per_switching_state)
  q_phase_voltage_per_switching_state3/1 -> Subsystem12/6(q_phase_voltage_per_switching_state)
  Subsystem8/1(id_8) -> Mux8/1
  Subsystem8/3(ix_8) -> Mux8/3
  Subsystem8/2(iq_8) -> Mux8/2
  Subsystem8/4(iy_8) -> Mux8/4
  Mux8/1 -> Prediction_8/1
  Subsystem9/1(id_7) -> Mux9/1
  Subsystem9/3(ix_7) -> Mux9/3
  Subsystem9/4(iy_7) -> Mux9/4
  Subsystem9/2(iq_7) -> Mux9/2
  Mux9/1 -> Prediction_7/1
  Subsystem10/4(iy_6) -> Mux10/4
  Subsystem10/2(iq_6) -> Mux10/2
  Subsystem10/3(ix_6) -> Mux10/3
  Subsystem10/1(id_6) -> Mux10/1
  Mux10/1 -> Prediction_6/1
  Subsystem11/3(ix_5) -> Mux11/3
  Subsystem11/4(iy_5) -> Mux11/4
  Subsystem11/2(iq_5) -> Mux11/2
  Subsystem11/1(id_5) -> Mux11/1
  Mux11/1 -> Prediction_5/1
  Subsystem12/4(iy_4) -> Mux12/4
  Subsystem12/2(iq_4) -> Mux12/2
  Mux12/1 -> Prediction_4/1
  Subsystem12/3(ix_4) -> Mux12/3
  Subsystem12/1(id_4) -> Mux12/1
  Subsystem13/2(iq_3) -> Mux13/2
  Subsystem13/4(iy_3) -> Mux13/4
  Subsystem13/3(ix_3) -> Mux13/3
  Subsystem13/1(id_3) -> Mux13/1
  Mux13/1 -> Prediction_3/1
  Subsystem14/1(id_2) -> Mux14/1
  Subsystem14/3(ix_2) -> Mux14/3
  Subsystem14/2(iq_2) -> Mux14/2
  Subsystem14/4(iy_2) -> Mux14/4
  Mux14/1 -> Prediction_2/1
  Subsystem15/4(iy_1) -> Mux15/4
  Subsystem15/2(iq_1) -> Mux15/2
  Subsystem15/1(id_1) -> Mux15/1
  Subsystem15/3(ix_1) -> Mux15/3
  Mux15/1 -> Prediction_1/1
  SampleTime_div_Ld15/1 -> Subsystem15/1(SampleTime_div_Ld), Subsystem8/1(SampleTime_div_Ld), Subsystem9/1(SampleTime_div_Ld), Subsystem10/1(SampleTime_div_Ld), Subsystem11/1(SampleTime_div_Ld), Subsystem12/1(SampleTime_div_Ld), Subsystem13/1(SampleTime_div_Ld), Subsystem14/1(SampleTime_div_Ld)  "SampleTime_div_Ld"
  SampleTime_div_Lq15/1 -> Subsystem8/2(SampleTime_div_Lq), Subsystem9/2(SampleTime_div_Lq), Subsystem10/2(SampleTime_div_Lq), Subsystem11/2(SampleTime_div_Lq), Subsystem12/2(SampleTime_div_Lq), Subsystem13/2(SampleTime_div_Lq), Subsystem14/2(SampleTime_div_Lq), Subsystem15/2(SampleTime_div_Lq)  "SampleTime_div_Lq"
  SampleTime_div_Lx15/1 -> Subsystem8/3(SampleTime_div_Lx), Subsystem9/3(SampleTime_div_Lx), Subsystem10/3(SampleTime_div_Lx), Subsystem11/3(SampleTime_div_Lx), Subsystem12/3(SampleTime_div_Lx), Subsystem13/3(SampleTime_div_Lx), Subsystem14/3(SampleTime_div_Lx), Subsystem15/3(SampleTime_div_Lx)  "SampleTime_div_Lx"
  SampleTime_div_Ly15/1 -> Subsystem8/4(SampleTime_div_Ly), Subsystem9/4(SampleTime_div_Ly), Subsystem10/4(SampleTime_div_Ly), Subsystem11/4(SampleTime_div_Ly), Subsystem12/4(SampleTime_div_Ly), Subsystem13/4(SampleTime_div_Ly), Subsystem14/4(SampleTime_div_Ly), Subsystem15/4(SampleTime_div_Ly)  "SampleTime_div_Ly"
  id_k_16/1 -> Subsystem8/9(id_k), Subsystem9/9(id_k), Subsystem10/9(id_k), Subsystem11/9(id_k), Subsystem12/9(id_k), Subsystem13/9(id_k), Subsystem14/9(id_k), Subsystem15/9(id_k)  "id_k"
  iq_k_16/1 -> Subsystem8/10(iq_k), Subsystem9/10(iq_k), Subsystem10/10(iq_k), Subsystem11/10(iq_k), Subsystem12/10(iq_k), Subsystem13/10(iq_k), Subsystem14/10(iq_k), Subsystem15/10(iq_k)  "iq_k"
  ix_k_16/1 -> Subsystem8/11(ix_k), Subsystem9/11(ix_k), Subsystem10/11(ix_k), Subsystem11/11(ix_k), Subsystem12/11(ix_k), Subsystem13/11(ix_k), Subsystem14/11(ix_k), Subsystem15/11(ix_k)  "ix_k"
  iy_k_16/1 -> Subsystem8/12(iy_k), Subsystem9/12(iy_k), Subsystem10/12(iy_k), Subsystem11/12(iy_k), Subsystem12/12(iy_k), Subsystem13/12(iy_k), Subsystem14/12(iy_k), Subsystem15/12(iy_k)  "iy_k"
  psiPM15/1 -> Subsystem14/13(psiPM), Subsystem8/13(psiPM), Subsystem9/13(psiPM), Subsystem10/13(psiPM), Subsystem11/13(psiPM), Subsystem12/13(psiPM), Subsystem13/13(psiPM), Subsystem15/13(psiPM)  "psiPM"
  Lq15/1 -> Subsystem8/14(Lq), Subsystem9/14(Lq), Subsystem10/14(Lq), Subsystem11/14(Lq), Subsystem12/14(Lq), Subsystem13/14(Lq), Subsystem14/14(Lq), Subsystem15/14(Lq)  "Lq"
  Ld15/1 -> Subsystem8/15(Ld), Subsystem9/15(Ld), Subsystem10/15(Ld), Subsystem11/15(Ld), Subsystem12/15(Ld), Subsystem13/15(Ld), Subsystem14/15(Ld), Subsystem15/15(Ld)  "Ld"
  Rs15/1 -> Subsystem8/16(Rs), Subsystem9/16(Rs), Subsystem10/16(Rs), Subsystem11/16(Rs), Subsystem12/16(Rs), Subsystem13/16(Rs), Subsystem14/16(Rs), Subsystem15/16(Rs)  "Rs"
  omega_el15/1 -> Subsystem8/17(omega_el), Subsystem9/17(omega_el), Subsystem10/17(omega_el), Subsystem11/17(omega_el), Subsystem12/17(omega_el), Subsystem13/17(omega_el), Subsystem14/17(omega_el), Subsystem15/17(omega_el)  "omega_el"

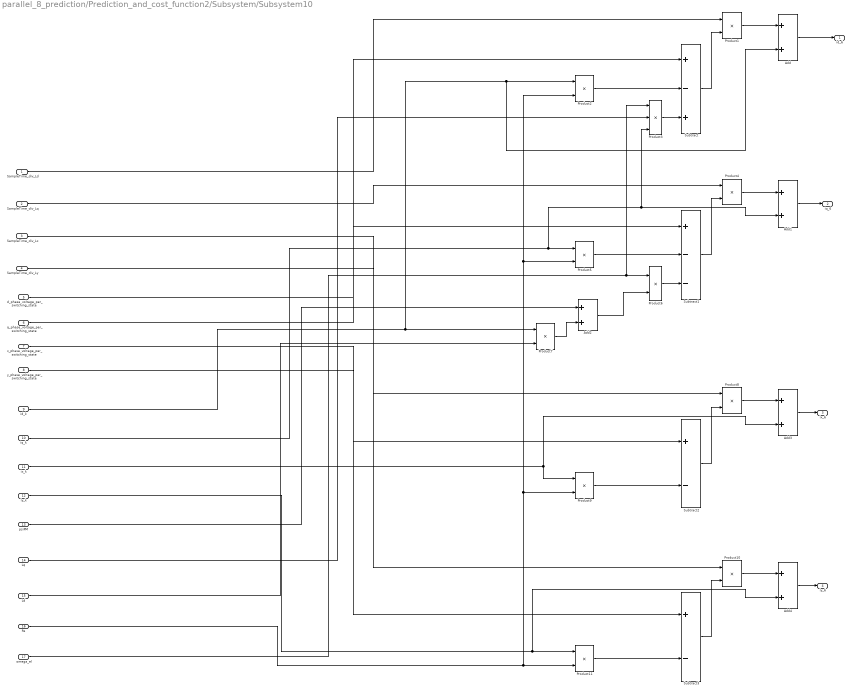
== system parallel_8_prediction/Prediction_and_cost_function2/Subsystem/Subsystem10 ==
  SampleTime_div_Ld : Inport
  SampleTime_div_Lq : Inport  Port=2
  SampleTime_div_Lx : Inport  Port=3
  SampleTime_div_Ly : Inport  Port=4
  d_phase_voltage_per_switching_state : Inport  Port=5
  q_phase_voltage_per_switching_state : Inport  Port=6
  x_phase_voltage_per_switching_state : Inport  Port=7
  y_phase_voltage_per_switching_state : Inport  Port=8
  id_k : Inport  Port=9
  iq_k : Inport  Port=10
  ix_k : Inport  Port=11
  iy_k : Inport  Port=12
  psiPM : Inport  Port=13
  Lq : Inport  Port=14
  Ld : Inport  Port=15
  Rs : Inport  Port=16
  omega_el : Inport  Port=17
  Add{,1,3..4} (4 alike) : Sum  OutDataTypeStr=single
  Add2 : Sum
  Product{1..2,4..11} (10 alike) : Product  OutDataTypeStr=single
  Product3 : Product  Inputs=3  OutDataTypeStr=single
  Subtract : Sum  Inputs=+-+  OutDataTypeStr=single
  Subtract1 : Sum  Inputs=+--  OutDataTypeStr=single
  Subtract2 : Sum  Inputs=+-  OutDataTypeStr=single
  Subtract3 : Sum  Inputs=+-  OutDataTypeStr=single
  id_6 : Outport
  iq_6 : Outport  Port=2
  ix_6 : Outport  Port=3
  iy_6 : Outport  Port=4
  wires:
  q_phase_voltage_per_switching_state/1 -> Subtract1/1
  omega_el/1 -> Product3/1, Product6/1
  Product5/1 -> Subtract1/2
  iq_k/1 -> Product3/3, Add1/2, Product5/1
  iy_k/1 -> Add4/2, Product11/1
  Add2/1 -> Product6/2
  Lq/1 -> Product3/2
  Subtract2/1 -> Product8/2
  SampleTime_div_Ly/1 -> Product10/1
  Rs/1 -> Product9/2, Product2/2, Product5/2, Product11/2
  Product9/1 -> Subtract2/2
  Product8/1 -> Add3/1
  Product7/1 -> Add2/2
  id_k/1 -> Add/2, Product2/1, Product7/1
  x_phase_voltage_per_switching_state/1 -> Subtract2/1
  Product11/1 -> Subtract3/2
  Product6/1 -> Subtract1/3
  Subtract1/1 -> Product4/2
  Product1/1 -> Add/1
  Product10/1 -> Add4/1
  Product4/1 -> Add1/1
  SampleTime_div_Ld/1 -> Product1/1
  y_phase_voltage_per_switching_state/1 -> Subtract3/1
  Product2/1 -> Subtract/2
  Product3/1 -> Subtract/3
  SampleTime_div_Lq/1 -> Product4/1
  Subtract/1 -> Product1/2
  Subtract3/1 -> Product10/2
  psiPM/1 -> Add2/1
  Ld/1 -> Product7/2
  ix_k/1 -> Add3/2, Product9/1
  SampleTime_div_Lx/1 -> Product8/1
  d_phase_voltage_per_switching_state/1 -> Subtract/1
  Add/1 -> id_6/1
  Add1/1 -> iq_6/1
  Add3/1 -> ix_6/1
  Add4/1 -> iy_6/1

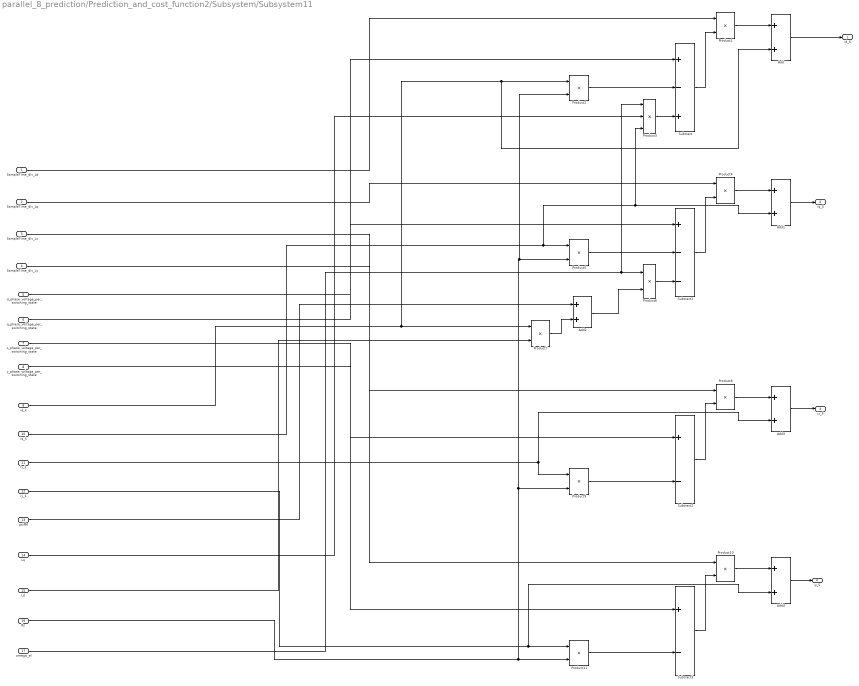
== system parallel_8_prediction/Prediction_and_cost_function2/Subsystem/Subsystem11 ==
  SampleTime_div_Ld : Inport
  SampleTime_div_Lq : Inport  Port=2
  SampleTime_div_Lx : Inport  Port=3
  SampleTime_div_Ly : Inport  Port=4
  d_phase_voltage_per_switching_state : Inport  Port=5
  q_phase_voltage_per_switching_state : Inport  Port=6
  x_phase_voltage_per_switching_state : Inport  Port=7
  y_phase_voltage_per_switching_state : Inport  Port=8
  id_k : Inport  Port=9
  iq_k : Inport  Port=10
  ix_k : Inport  Port=11
  iy_k : Inport  Port=12
  psiPM : Inport  Port=13
  Lq : Inport  Port=14
  Ld : Inport  Port=15
  Rs : Inport  Port=16
  omega_el : Inport  Port=17
  Add{,1,3..4} (4 alike) : Sum  OutDataTypeStr=single
  Add2 : Sum
  Product{1..2,4..11} (10 alike) : Product  OutDataTypeStr=single
  Product3 : Product  Inputs=3  OutDataTypeStr=single
  Subtract : Sum  Inputs=+-+  OutDataTypeStr=single
  Subtract1 : Sum  Inputs=+--  OutDataTypeStr=single
  Subtract2 : Sum  Inputs=+-  OutDataTypeStr=single
  Subtract3 : Sum  Inputs=+-  OutDataTypeStr=single
  id_5 : Outport
  iq_5 : Outport  Port=2
  ix_5 : Outport  Port=3
  iy_5 : Outport  Port=4
  wires:
  q_phase_voltage_per_switching_state/1 -> Subtract1/1
  omega_el/1 -> Product3/1, Product6/1
  Product5/1 -> Subtract1/2
  iq_k/1 -> Product3/3, Add1/2, Product5/1
  iy_k/1 -> Add4/2, Product11/1
  Add2/1 -> Product6/2
  Lq/1 -> Product3/2
  Subtract2/1 -> Product8/2
  SampleTime_div_Ly/1 -> Product10/1
  Rs/1 -> Product9/2, Product2/2, Product5/2, Product11/2
  Product9/1 -> Subtract2/2
  Product8/1 -> Add3/1
  Product7/1 -> Add2/2
  id_k/1 -> Add/2, Product2/1, Product7/1
  x_phase_voltage_per_switching_state/1 -> Subtract2/1
  Product11/1 -> Subtract3/2
  Product6/1 -> Subtract1/3
  Subtract1/1 -> Product4/2
  Product1/1 -> Add/1
  Product10/1 -> Add4/1
  Product4/1 -> Add1/1
  SampleTime_div_Ld/1 -> Product1/1
  y_phase_voltage_per_switching_state/1 -> Subtract3/1
  Product2/1 -> Subtract/2
  Product3/1 -> Subtract/3
  SampleTime_div_Lq/1 -> Product4/1
  Subtract/1 -> Product1/2
  Subtract3/1 -> Product10/2
  psiPM/1 -> Add2/1
  Ld/1 -> Product7/2
  ix_k/1 -> Add3/2, Product9/1
  SampleTime_div_Lx/1 -> Product8/1
  d_phase_voltage_per_switching_state/1 -> Subtract/1
  Add/1 -> id_5/1
  Add1/1 -> iq_5/1
  Add3/1 -> ix_5/1
  Add4/1 -> iy_5/1

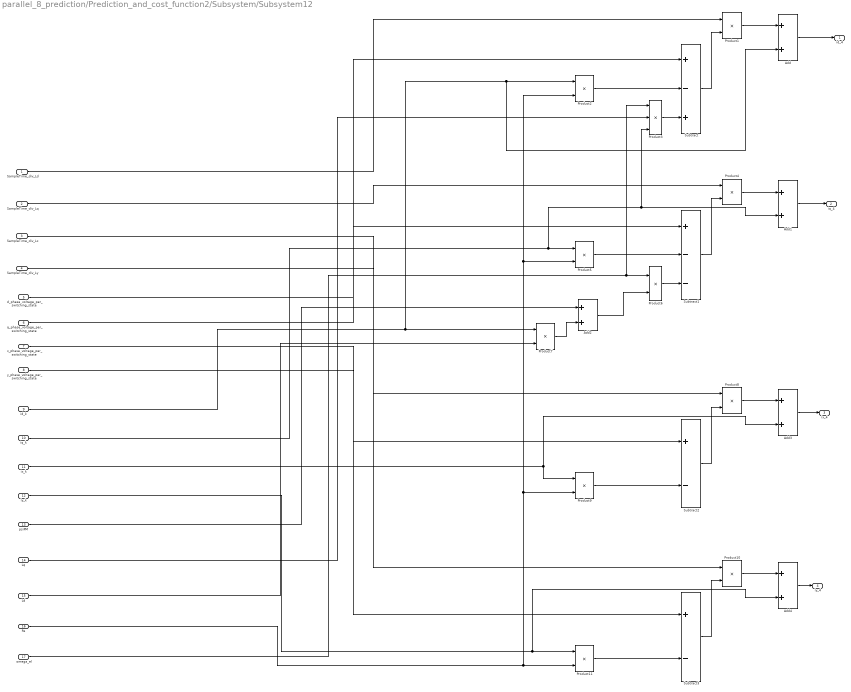
== system parallel_8_prediction/Prediction_and_cost_function2/Subsystem/Subsystem12 ==
  SampleTime_div_Ld : Inport
  SampleTime_div_Lq : Inport  Port=2
  SampleTime_div_Lx : Inport  Port=3
  SampleTime_div_Ly : Inport  Port=4
  d_phase_voltage_per_switching_state : Inport  Port=5
  q_phase_voltage_per_switching_state : Inport  Port=6
  x_phase_voltage_per_switching_state : Inport  Port=7
  y_phase_voltage_per_switching_state : Inport  Port=8
  id_k : Inport  Port=9
  iq_k : Inport  Port=10
  ix_k : Inport  Port=11
  iy_k : Inport  Port=12
  psiPM : Inport  Port=13
  Lq : Inport  Port=14
  Ld : Inport  Port=15
  Rs : Inport  Port=16
  omega_el : Inport  Port=17
  Add{,1,3..4} (4 alike) : Sum  OutDataTypeStr=single
  Add2 : Sum
  Product{1..2,4..11} (10 alike) : Product  OutDataTypeStr=single
  Product3 : Product  Inputs=3  OutDataTypeStr=single
  Subtract : Sum  Inputs=+-+  OutDataTypeStr=single
  Subtract1 : Sum  Inputs=+--  OutDataTypeStr=single
  Subtract2 : Sum  Inputs=+-  OutDataTypeStr=single
  Subtract3 : Sum  Inputs=+-  OutDataTypeStr=single
  id_4 : Outport
  iq_4 : Outport  Port=2
  ix_4 : Outport  Port=3
  iy_4 : Outport  Port=4
  wires:
  q_phase_voltage_per_switching_state/1 -> Subtract1/1
  omega_el/1 -> Product3/1, Product6/1
  Product5/1 -> Subtract1/2
  iq_k/1 -> Product3/3, Add1/2, Product5/1
  iy_k/1 -> Add4/2, Product11/1
  Add2/1 -> Product6/2
  Lq/1 -> Product3/2
  Subtract2/1 -> Product8/2
  SampleTime_div_Ly/1 -> Product10/1
  Rs/1 -> Product9/2, Product2/2, Product5/2, Product11/2
  Product9/1 -> Subtract2/2
  Product8/1 -> Add3/1
  Product7/1 -> Add2/2
  id_k/1 -> Add/2, Product2/1, Product7/1
  x_phase_voltage_per_switching_state/1 -> Subtract2/1
  Product11/1 -> Subtract3/2
  Product6/1 -> Subtract1/3
  Subtract1/1 -> Product4/2
  Product1/1 -> Add/1
  Product10/1 -> Add4/1
  Product4/1 -> Add1/1
  SampleTime_div_Ld/1 -> Product1/1
  y_phase_voltage_per_switching_state/1 -> Subtract3/1
  Product2/1 -> Subtract/2
  Product3/1 -> Subtract/3
  SampleTime_div_Lq/1 -> Product4/1
  Subtract/1 -> Product1/2
  Subtract3/1 -> Product10/2
  psiPM/1 -> Add2/1
  Ld/1 -> Product7/2
  ix_k/1 -> Add3/2, Product9/1
  SampleTime_div_Lx/1 -> Product8/1
  d_phase_voltage_per_switching_state/1 -> Subtract/1
  Add/1 -> id_4/1
  Add1/1 -> iq_4/1
  Add3/1 -> ix_4/1
  Add4/1 -> iy_4/1

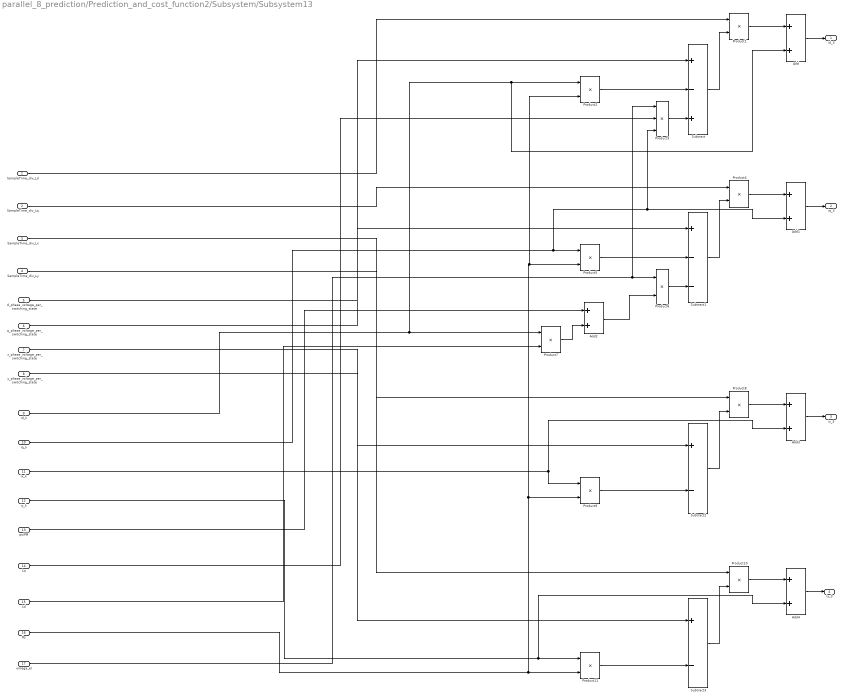
== system parallel_8_prediction/Prediction_and_cost_function2/Subsystem/Subsystem13 ==
  SampleTime_div_Ld : Inport
  SampleTime_div_Lq : Inport  Port=2
  SampleTime_div_Lx : Inport  Port=3
  SampleTime_div_Ly : Inport  Port=4
  d_phase_voltage_per_switching_state : Inport  Port=5
  q_phase_voltage_per_switching_state : Inport  Port=6
  x_phase_voltage_per_switching_state : Inport  Port=7
  y_phase_voltage_per_switching_state : Inport  Port=8
  id_k : Inport  Port=9
  iq_k : Inport  Port=10
  ix_k : Inport  Port=11
  iy_k : Inport  Port=12
  psiPM : Inport  Port=13
  Lq : Inport  Port=14
  Ld : Inport  Port=15
  Rs : Inport  Port=16
  omega_el : Inport  Port=17
  Add{,1,3..4} (4 alike) : Sum  OutDataTypeStr=single
  Add2 : Sum
  Product{1..2,4..11} (10 alike) : Product  OutDataTypeStr=single
  Product3 : Product  Inputs=3  OutDataTypeStr=single
  Subtract : Sum  Inputs=+-+  OutDataTypeStr=single
  Subtract1 : Sum  Inputs=+--  OutDataTypeStr=single
  Subtract2 : Sum  Inputs=+-  OutDataTypeStr=single
  Subtract3 : Sum  Inputs=+-  OutDataTypeStr=single
  id_3 : Outport
  iq_3 : Outport  Port=2
  ix_3 : Outport  Port=3
  iy_3 : Outport  Port=4
  wires:
  q_phase_voltage_per_switching_state/1 -> Subtract1/1
  omega_el/1 -> Product3/1, Product6/1
  Product5/1 -> Subtract1/2
  iq_k/1 -> Product3/3, Add1/2, Product5/1
  iy_k/1 -> Add4/2, Product11/1
  Add2/1 -> Product6/2
  Lq/1 -> Product3/2
  Subtract2/1 -> Product8/2
  SampleTime_div_Ly/1 -> Product10/1
  Rs/1 -> Product9/2, Product2/2, Product5/2, Product11/2
  Product9/1 -> Subtract2/2
  Product8/1 -> Add3/1
  Product7/1 -> Add2/2
  id_k/1 -> Add/2, Product2/1, Product7/1
  x_phase_voltage_per_switching_state/1 -> Subtract2/1
  Product11/1 -> Subtract3/2
  Product6/1 -> Subtract1/3
  Subtract1/1 -> Product4/2
  Product1/1 -> Add/1
  Product10/1 -> Add4/1
  Product4/1 -> Add1/1
  SampleTime_div_Ld/1 -> Product1/1
  y_phase_voltage_per_switching_state/1 -> Subtract3/1
  Product2/1 -> Subtract/2
  Product3/1 -> Subtract/3
  SampleTime_div_Lq/1 -> Product4/1
  Subtract/1 -> Product1/2
  Subtract3/1 -> Product10/2
  psiPM/1 -> Add2/1
  Ld/1 -> Product7/2
  ix_k/1 -> Add3/2, Product9/1
  SampleTime_div_Lx/1 -> Product8/1
  d_phase_voltage_per_switching_state/1 -> Subtract/1
  Add/1 -> id_3/1
  Add1/1 -> iq_3/1
  Add3/1 -> ix_3/1
  Add4/1 -> iy_3/1

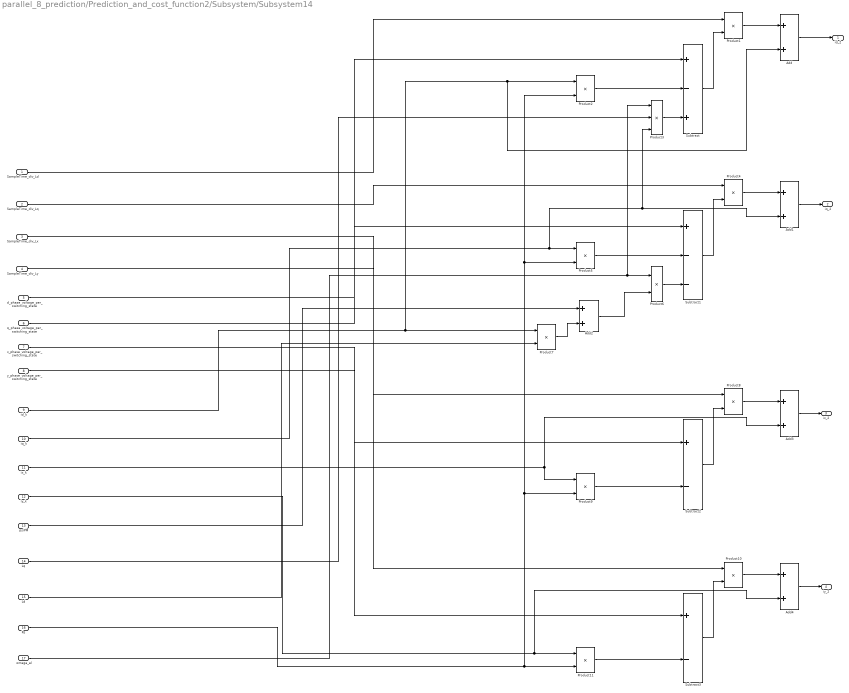
== system parallel_8_prediction/Prediction_and_cost_function2/Subsystem/Subsystem14 ==
  SampleTime_div_Ld : Inport
  SampleTime_div_Lq : Inport  Port=2
  SampleTime_div_Lx : Inport  Port=3
  SampleTime_div_Ly : Inport  Port=4
  d_phase_voltage_per_switching_state : Inport  Port=5
  q_phase_voltage_per_switching_state : Inport  Port=6
  x_phase_voltage_per_switching_state : Inport  Port=7
  y_phase_voltage_per_switching_state : Inport  Port=8
  id_k : Inport  Port=9
  iq_k : Inport  Port=10
  ix_k : Inport  Port=11
  iy_k : Inport  Port=12
  psiPM : Inport  Port=13
  Lq : Inport  Port=14
  Ld : Inport  Port=15
  Rs : Inport  Port=16
  omega_el : Inport  Port=17
  Add{,1,3..4} (4 alike) : Sum  OutDataTypeStr=single
  Add2 : Sum
  Product{1..2,4..11} (10 alike) : Product  OutDataTypeStr=single
  Product3 : Product  Inputs=3  OutDataTypeStr=single
  Subtract : Sum  Inputs=+-+  OutDataTypeStr=single
  Subtract1 : Sum  Inputs=+--  OutDataTypeStr=single
  Subtract2 : Sum  Inputs=+-  OutDataTypeStr=single
  Subtract3 : Sum  Inputs=+-  OutDataTypeStr=single
  id_2 : Outport
  iq_2 : Outport  Port=2
  ix_2 : Outport  Port=3
  iy_2 : Outport  Port=4
  wires:
  q_phase_voltage_per_switching_state/1 -> Subtract1/1
  omega_el/1 -> Product3/1, Product6/1
  Product5/1 -> Subtract1/2
  iq_k/1 -> Product3/3, Add1/2, Product5/1
  iy_k/1 -> Add4/2, Product11/1
  Add2/1 -> Product6/2
  Lq/1 -> Product3/2
  Subtract2/1 -> Product8/2
  SampleTime_div_Ly/1 -> Product10/1
  Rs/1 -> Product9/2, Product2/2, Product5/2, Product11/2
  Product9/1 -> Subtract2/2
  Product8/1 -> Add3/1
  Product7/1 -> Add2/2
  id_k/1 -> Add/2, Product2/1, Product7/1
  x_phase_voltage_per_switching_state/1 -> Subtract2/1
  Product11/1 -> Subtract3/2
  Product6/1 -> Subtract1/3
  Subtract1/1 -> Product4/2
  Product1/1 -> Add/1
  Product10/1 -> Add4/1
  Product4/1 -> Add1/1
  SampleTime_div_Ld/1 -> Product1/1
  y_phase_voltage_per_switching_state/1 -> Subtract3/1
  Product2/1 -> Subtract/2
  Product3/1 -> Subtract/3
  SampleTime_div_Lq/1 -> Product4/1
  Subtract/1 -> Product1/2
  Subtract3/1 -> Product10/2
  psiPM/1 -> Add2/1
  Ld/1 -> Product7/2
  ix_k/1 -> Add3/2, Product9/1
  SampleTime_div_Lx/1 -> Product8/1
  d_phase_voltage_per_switching_state/1 -> Subtract/1
  Add/1 -> id_2/1
  Add1/1 -> iq_2/1
  Add3/1 -> ix_2/1
  Add4/1 -> iy_2/1

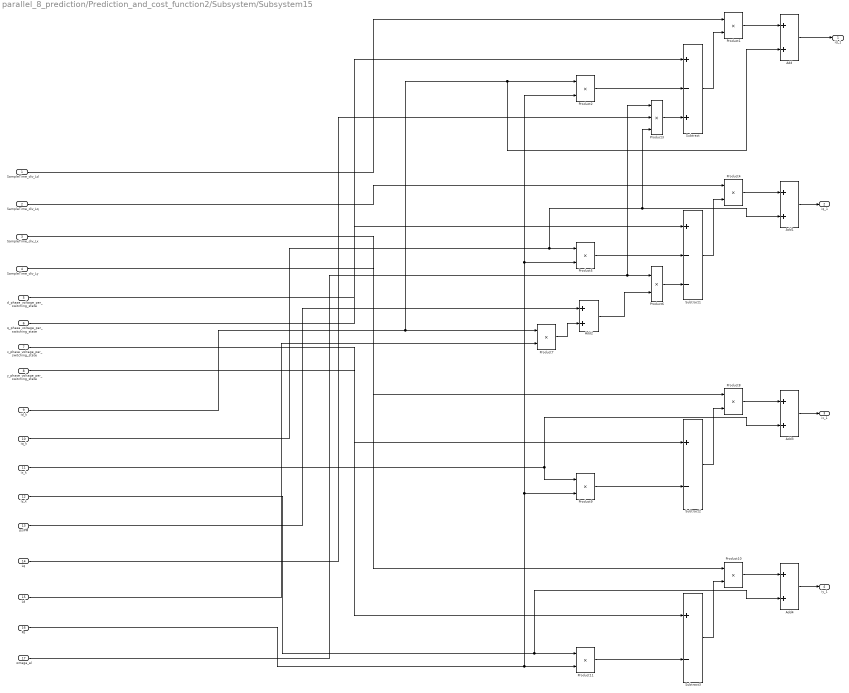
== system parallel_8_prediction/Prediction_and_cost_function2/Subsystem/Subsystem15 ==
  SampleTime_div_Ld : Inport
  SampleTime_div_Lq : Inport  Port=2
  SampleTime_div_Lx : Inport  Port=3
  SampleTime_div_Ly : Inport  Port=4
  d_phase_voltage_per_switching_state : Inport  Port=5
  q_phase_voltage_per_switching_state : Inport  Port=6
  x_phase_voltage_per_switching_state : Inport  Port=7
  y_phase_voltage_per_switching_state : Inport  Port=8
  id_k : Inport  Port=9
  iq_k : Inport  Port=10
  ix_k : Inport  Port=11
  iy_k : Inport  Port=12
  psiPM : Inport  Port=13
  Lq : Inport  Port=14
  Ld : Inport  Port=15
  Rs : Inport  Port=16
  omega_el : Inport  Port=17
  Add{,1,3..4} (4 alike) : Sum  OutDataTypeStr=single
  Add2 : Sum
  Product{1..2,4..11} (10 alike) : Product  OutDataTypeStr=single
  Product3 : Product  Inputs=3  OutDataTypeStr=single
  Subtract : Sum  Inputs=+-+  OutDataTypeStr=single
  Subtract1 : Sum  Inputs=+--  OutDataTypeStr=single
  Subtract2 : Sum  Inputs=+-  OutDataTypeStr=single
  Subtract3 : Sum  Inputs=+-  OutDataTypeStr=single
  id_1 : Outport
  iq_1 : Outport  Port=2
  ix_1 : Outport  Port=3
  iy_1 : Outport  Port=4
  wires:
  q_phase_voltage_per_switching_state/1 -> Subtract1/1
  omega_el/1 -> Product3/1, Product6/1
  Product5/1 -> Subtract1/2
  iq_k/1 -> Product3/3, Add1/2, Product5/1
  iy_k/1 -> Add4/2, Product11/1
  Add2/1 -> Product6/2
  Lq/1 -> Product3/2
  Subtract2/1 -> Product8/2
  SampleTime_div_Ly/1 -> Product10/1
  Rs/1 -> Product9/2, Product2/2, Product5/2, Product11/2
  Product9/1 -> Subtract2/2
  Product8/1 -> Add3/1
  Product7/1 -> Add2/2
  id_k/1 -> Add/2, Product2/1, Product7/1
  x_phase_voltage_per_switching_state/1 -> Subtract2/1
  Product11/1 -> Subtract3/2
  Product6/1 -> Subtract1/3
  Subtract1/1 -> Product4/2
  Product1/1 -> Add/1
  Product10/1 -> Add4/1
  Product4/1 -> Add1/1
  SampleTime_div_Ld/1 -> Product1/1
  y_phase_voltage_per_switching_state/1 -> Subtract3/1
  Product2/1 -> Subtract/2
  Product3/1 -> Subtract/3
  SampleTime_div_Lq/1 -> Product4/1
  Subtract/1 -> Product1/2
  Subtract3/1 -> Product10/2
  psiPM/1 -> Add2/1
  Ld/1 -> Product7/2
  ix_k/1 -> Add3/2, Product9/1
  SampleTime_div_Lx/1 -> Product8/1
  d_phase_voltage_per_switching_state/1 -> Subtract/1
  Add/1 -> id_1/1
  Add1/1 -> iq_1/1
  Add3/1 -> ix_1/1
  Add4/1 -> iy_1/1

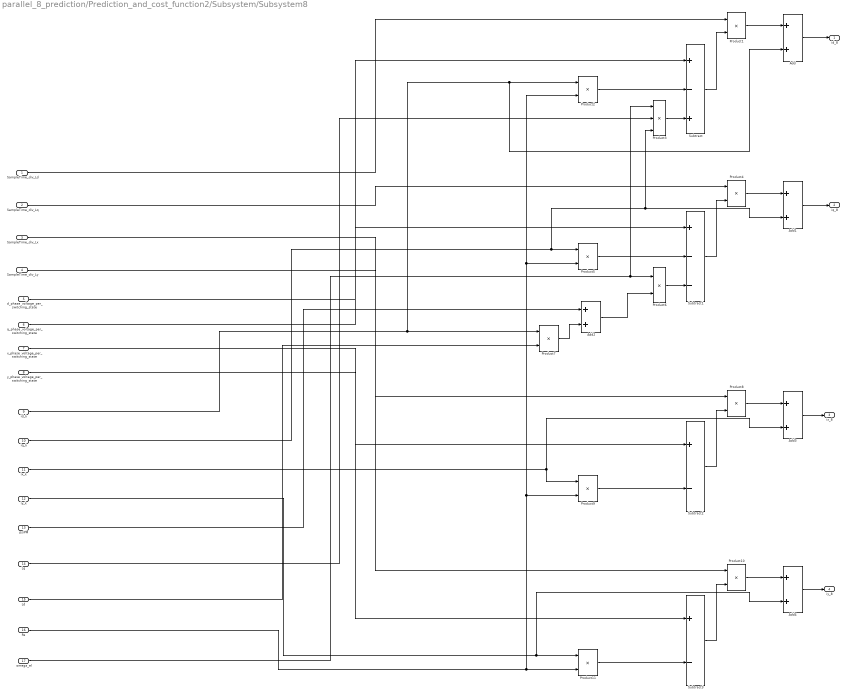
== system parallel_8_prediction/Prediction_and_cost_function2/Subsystem/Subsystem8 ==
  SampleTime_div_Ld : Inport
  SampleTime_div_Lq : Inport  Port=2
  SampleTime_div_Lx : Inport  Port=3
  SampleTime_div_Ly : Inport  Port=4
  d_phase_voltage_per_switching_state : Inport  Port=5
  q_phase_voltage_per_switching_state : Inport  Port=6
  x_phase_voltage_per_switching_state : Inport  Port=7
  y_phase_voltage_per_switching_state : Inport  Port=8
  id_k : Inport  Port=9
  iq_k : Inport  Port=10
  ix_k : Inport  Port=11
  iy_k : Inport  Port=12
  psiPM : Inport  Port=13
  Lq : Inport  Port=14
  Ld : Inport  Port=15
  Rs : Inport  Port=16
  omega_el : Inport  Port=17
  Add{,1,3..4} (4 alike) : Sum  OutDataTypeStr=single
  Add2 : Sum
  Product{1..2,4..11} (10 alike) : Product  OutDataTypeStr=single
  Product3 : Product  Inputs=3  OutDataTypeStr=single
  Subtract : Sum  Inputs=+-+  OutDataTypeStr=single
  Subtract1 : Sum  Inputs=+--  OutDataTypeStr=single
  Subtract2 : Sum  Inputs=+-  OutDataTypeStr=single
  Subtract3 : Sum  Inputs=+-  OutDataTypeStr=single
  id_8 : Outport
  iq_8 : Outport  Port=2
  ix_8 : Outport  Port=3
  iy_8 : Outport  Port=4
  wires:
  q_phase_voltage_per_switching_state/1 -> Subtract1/1
  omega_el/1 -> Product3/1, Product6/1
  Product5/1 -> Subtract1/2
  iq_k/1 -> Product3/3, Add1/2, Product5/1
  iy_k/1 -> Add4/2, Product11/1
  Add2/1 -> Product6/2
  Lq/1 -> Product3/2
  Subtract2/1 -> Product8/2
  SampleTime_div_Ly/1 -> Product10/1
  Rs/1 -> Product9/2, Product2/2, Product5/2, Product11/2
  Product9/1 -> Subtract2/2
  Product8/1 -> Add3/1
  Product7/1 -> Add2/2
  id_k/1 -> Add/2, Product2/1, Product7/1
  x_phase_voltage_per_switching_state/1 -> Subtract2/1
  Product11/1 -> Subtract3/2
  Product6/1 -> Subtract1/3
  Subtract1/1 -> Product4/2
  Product1/1 -> Add/1
  Product10/1 -> Add4/1
  Product4/1 -> Add1/1
  SampleTime_div_Ld/1 -> Product1/1
  y_phase_voltage_per_switching_state/1 -> Subtract3/1
  Product2/1 -> Subtract/2
  Product3/1 -> Subtract/3
  SampleTime_div_Lq/1 -> Product4/1
  Subtract/1 -> Product1/2
  Subtract3/1 -> Product10/2
  psiPM/1 -> Add2/1
  Ld/1 -> Product7/2
  ix_k/1 -> Add3/2, Product9/1
  SampleTime_div_Lx/1 -> Product8/1
  d_phase_voltage_per_switching_state/1 -> Subtract/1
  Add/1 -> id_8/1
  Add1/1 -> iq_8/1
  Add3/1 -> ix_8/1
  Add4/1 -> iy_8/1
